simulink model "poisson2"  (R2023b)
settings: Solver=ode45  StartTime=0  StopTime=30  FixedStep=1  RelTol=1e-3
undefined symbols (not defined in the file): m, n
settings Model: Creator=anruk  LastModifiedBy=anruk

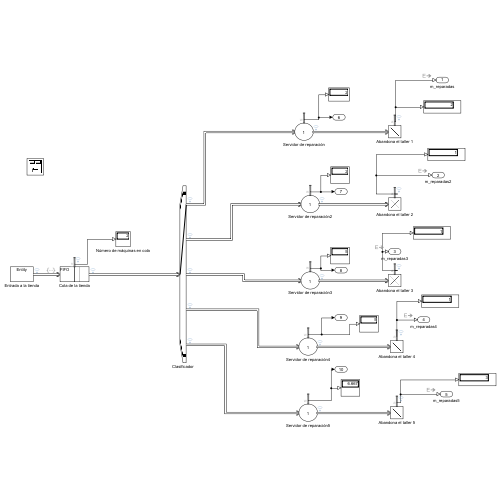
[thumbnail: Simulink's stored preview of the top-level diagram]
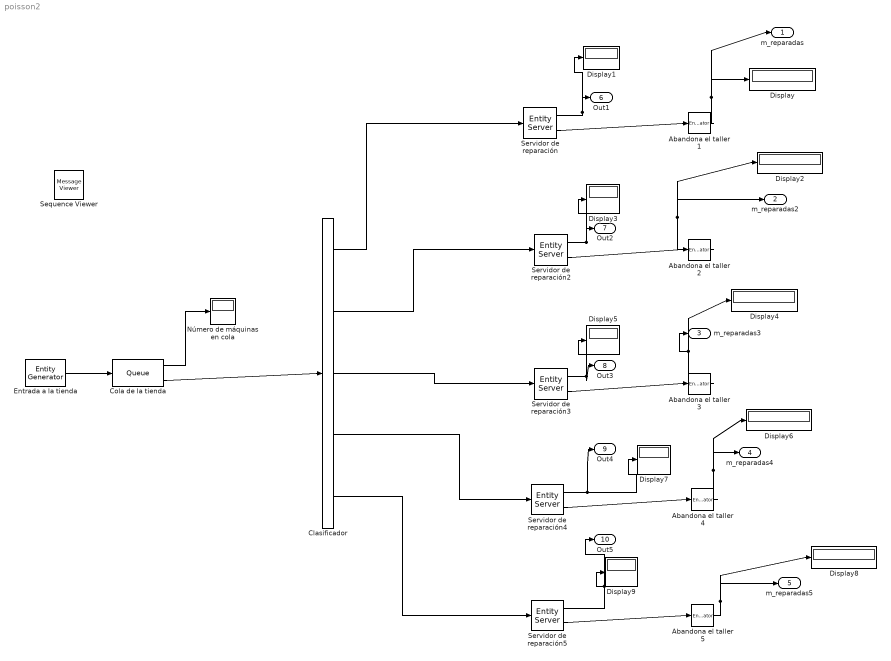
== system poisson2 ==
  Abandona el taller {1..5} (5 alike) : EntityTerminator  InputPortMessageModes=m  NumberEntitiesArrived=on
      settings: OutputPortMap=o0
  Clasificador : EntityOutputSwitch  InputPortMessageModes=m  OutputPortMessageModes=m,m,m,m,m  NumberOutputPorts=5  SwitchingCriterion=From attribute  SwitchAttributeName=MaquinaTipo
      settings: OutputPortMap=o0,o1,o2,o3,o4
  Cola de la tienda : Queue  InputPortMessageModes=m  OutputPortMessageModes=n,m  Capacity=10  EntryAction=entity.MaquinaTipo = randi([1,5]);  NumberEntitiesInBlock=on
      settings: OutputPortMap=o1,o5
  Display{,1..9} (10 alike) : Display
  Entrada a la tienda : EntityGenerator  OutputPortMessageModes=m  TimeSource=MATLAB action  IntergenerationTimeAction=|  GenerateEntityAtSimulationStart=off  AttributeName=MaquinaTipo  EntityType=Structured  EntityTypeName=Entity
      | % Distribucion de poisson con media 2
      | dt = poissrnd(2);
  Número de máquinas en cola : Display
  Sequence Viewer : MessageViewer  History=1000  SavedRootId=#
  Servidor de reparación : EntityServer  InputPortMessageModes=m  OutputPortMessageModes=n,m  Capacity=1  ServiceTimeSource=MATLAB action  ServiceTimeAction=|  AverageWait=on
      | % Distribucion de poisson con media 1,2,3,4 o 5 
      | % Dependiendo del tipo de máquina
      | dt = poissrnd(entity.MaquinaTipo);
      settings: OutputPortMap=o4,o9
  Servidor de reparación2 : EntityServer  InputPortMessageModes=m  OutputPortMessageModes=n,m  Capacity=1  ServiceTimeSource=MATLAB action  ServiceTimeAction=|  AverageWait=on
      | % Distribucion de poisson con media 1,2,3,4 o 5 
      | % Dependiendo del tipo de máquina
      | dt = poissrnd(entity.MaquinaTipo);
      settings: OutputPortMap=o4,o9
  Servidor de reparación3 : EntityServer  InputPortMessageModes=m  OutputPortMessageModes=n,m  Capacity=1  ServiceTimeSource=MATLAB action  ServiceTimeAction=|  AverageWait=on
      | % Distribucion de poisson con media 1,2,3,4 o 5 
      | % Dependiendo del tipo de máquina
      | dt = poissrnd(entity.MaquinaTipo);
      settings: OutputPortMap=o4,o9
  Servidor de reparación4 : EntityServer  InputPortMessageModes=m  OutputPortMessageModes=n,m  Capacity=1  ServiceTimeSource=MATLAB action  ServiceTimeAction=|  AverageWait=on
      | % Distribucion de poisson con media 1,2,3,4 o 5 
      | % Dependiendo del tipo de máquina
      | dt = poissrnd(entity.MaquinaTipo);
      settings: OutputPortMap=o4,o9
  Servidor de reparación5 : EntityServer  InputPortMessageModes=m  OutputPortMessageModes=n,m  Capacity=1  ServiceTimeSource=MATLAB action  ServiceTimeAction=|  AverageWait=on
      | % Distribucion de poisson con media 1,2,3,4 o 5 
      | % Dependiendo del tipo de máquina
      | dt = poissrnd(entity.MaquinaTipo);
      settings: OutputPortMap=o4,o9
  m_reparadas : Outport
  m_reparadas2 : Outport  Port=2
  m_reparadas3 : Outport  Port=3
  m_reparadas4 : Outport  Port=4
  m_reparadas5 : Outport  Port=5
  Out1 : Outport  Port=6
  Out2 : Outport  Port=7
  Out3 : Outport  Port=8
  Out4 : Outport  Port=9
  Out5 : Outport  Port=10
  wires:
  Entrada a la tienda/1 -> Cola de la tienda/1
  Servidor de reparación/2 -> Abandona el taller 1/1
  Abandona el taller 1/1 -> m_reparadas/1, Display/1
  Cola de la tienda/1 -> Número de máquinas en cola/1
  Cola de la tienda/2 -> Clasificador/1
  Clasificador/1 -> Servidor de reparación/1
  Clasificador/2 -> Servidor de reparación2/1
  Servidor de reparación2/2 -> Abandona el taller 2/1
  Abandona el taller 2/1 -> Display2/1, m_reparadas2/1
  Servidor de reparación2/1 -> Out2/1, Display3/1
  Clasificador/3 -> Servidor de reparación3/1
  Servidor de reparación3/2 -> Abandona el taller 3/1
  Abandona el taller 3/1 -> Display4/1, m_reparadas3/1
  Clasificador/4 -> Servidor de reparación4/1
  Abandona el taller 4/1 -> Display6/1, m_reparadas4/1
  Servidor de reparación4/2 -> Abandona el taller 4/1
  Clasificador/5 -> Servidor de reparación5/1
  Abandona el taller 5/1 -> Display8/1, m_reparadas5/1
  Servidor de reparación5/2 -> Abandona el taller 5/1
  Servidor de reparación5/1 -> Out5/1, Display9/1
  Servidor de reparación4/1 -> Out4/1, Display7/1
  Servidor de reparación3/1 -> Display5/1, Out3/1
  Servidor de reparación/1 -> Out1/1, Display1/1
